simulink model "inverted_pendulum"  (R2017b)
settings: Solver=FixedStepAuto  StartTime=0.0  StopTime=10  FixedStep=0.01  RelTol=1e-3
undefined symbols (not defined in the file or in its folder): gamma, Jt, k1, k2, len, mg, omega0, theta0
settings Model: Creator=tonypai  LastModifiedBy=tonypai
settings CodeAppCC: StateflowObjectComments=on

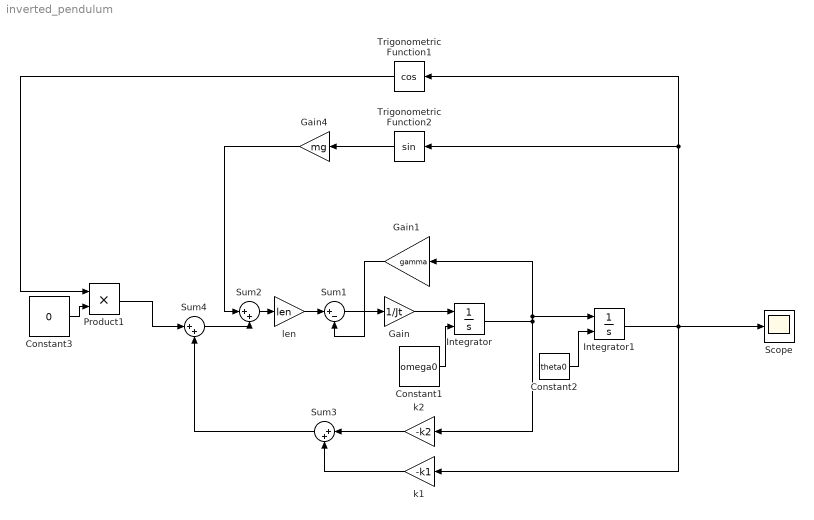
== system inverted_pendulum ==
  Constant1 : Constant  Value=omega0
  Constant2 : Constant  Value=theta0
  Constant3 : Constant  Value=0
  Gain : Gain  Gain=1/Jt
  Gain1 : Gain  Gain=gamma
  Gain4 : Gain  Gain=mg
  Integrator : Integrator  InitialConditionSource=external
  Integrator1 : Integrator  InitialConditionSource=external
  Product1 : Product
  Scope : Scope
  Sum1 : Sum  Inputs=|+-
  Sum2 : Sum  Inputs=|++
  Sum3 : Sum  Inputs=|++
  Sum4 : Sum  Inputs=|++
  Trigonometric Function1 : Trigonometry  Operator=cos
  Trigonometric Function2 : Trigonometry
  k1 : Gain  Gain=-k1
  k2 : Gain  Gain=-k2
  "len " : Gain  Gain=len
  wires:
  Trigonometric Function2/1 -> Gain4/1
  Gain4/1 -> Sum2/1
  "len "/1 -> Sum1/1
  Gain1/1 -> Sum1/2
  Sum1/1 -> Gain/1
  Gain/1 -> Integrator/1
  Constant1/1 -> Integrator/2
  Integrator1/1 -> k1/1, Trigonometric Function2/1, Trigonometric Function1/1, Scope/1
  Constant2/1 -> Integrator1/2
  Integrator/1 -> Gain1/1, Integrator1/1, k2/1
  k2/1 -> Sum3/1
  k1/1 -> Sum3/2
  Sum2/1 -> "len "/1
  Sum3/1 -> Sum4/2
  Trigonometric Function1/1 -> Product1/1
  Constant3/1 -> Product1/2
  Product1/1 -> Sum4/1
  Sum4/1 -> Sum2/2
